simulink model "TST_CoPT_TrqDesCoord"  (R2016b)
settings: Solver=FixedStepDiscrete  StartTime=0.0  StopTime=simTime  FixedStep=sampleTime  RelTol=1e-3
values from neighbouring files (symbols this model uses):
  testCase = 1    [initTST_CoPT_TrqDesCoord_001.m]    (also in initTST_CoPT_TrqDesCoord_002.m = 2; initTST_CoPT_TrqDesCoord_003.m = 3)
libraries: simulink x16, UnitTest_Lib x12
settings Model: Creator=zhengjinyan  LastModifiedBy=zhengjinyan
settings DebuggingCC: SignalRangeChecking=error

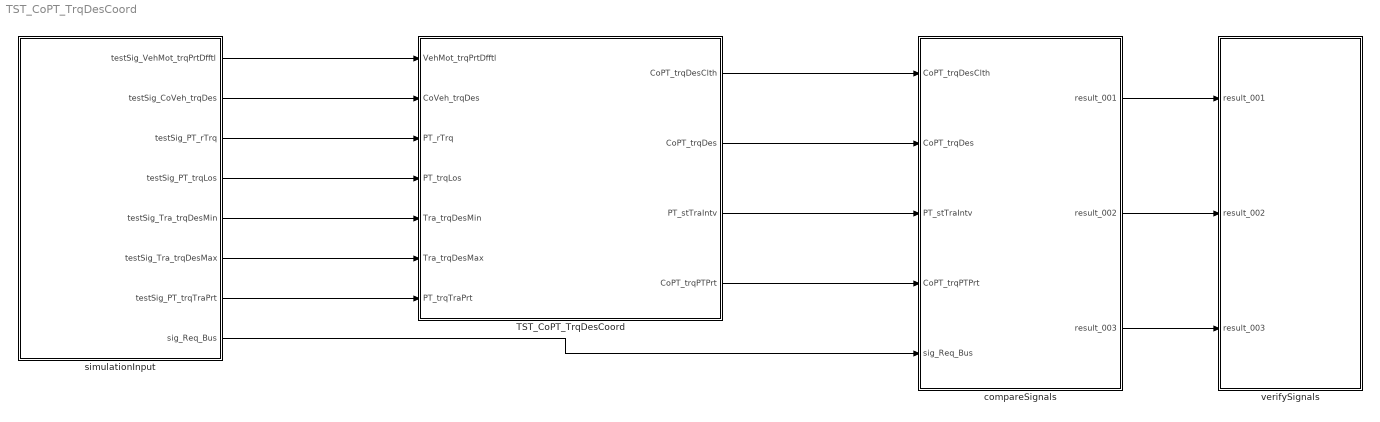
== system TST_CoPT_TrqDesCoord ==
  TST_CoPT_TrqDesCoord : Subsystem
  compareSignals : Subsystem
  simulationInput : Subsystem
  verifySignals : Subsystem
  wires:
  simulationInput/1(testSig_VehMot_trqPrtDfftl) -> TST_CoPT_TrqDesCoord/1(VehMot_trqPrtDfftl)
  simulationInput/2(testSig_CoVeh_trqDes) -> TST_CoPT_TrqDesCoord/2(CoVeh_trqDes)
  simulationInput/3(testSig_PT_rTrq) -> TST_CoPT_TrqDesCoord/3(PT_rTrq)
  simulationInput/4(testSig_PT_trqLos) -> TST_CoPT_TrqDesCoord/4(PT_trqLos)
  simulationInput/5(testSig_Tra_trqDesMin) -> TST_CoPT_TrqDesCoord/5(Tra_trqDesMin)
  simulationInput/6(testSig_Tra_trqDesMax) -> TST_CoPT_TrqDesCoord/6(Tra_trqDesMax)
  simulationInput/7(testSig_PT_trqTraPrt) -> TST_CoPT_TrqDesCoord/7(PT_trqTraPrt)
  TST_CoPT_TrqDesCoord/1(CoPT_trqDesClth) -> compareSignals/1(CoPT_trqDesClth)
  TST_CoPT_TrqDesCoord/2(CoPT_trqDes) -> compareSignals/2(CoPT_trqDes)
  TST_CoPT_TrqDesCoord/3(PT_stTraIntv) -> compareSignals/3(PT_stTraIntv)
  TST_CoPT_TrqDesCoord/4(CoPT_trqPTPrt) -> compareSignals/4(CoPT_trqPTPrt)
  simulationInput/8(sig_Req_Bus) -> compareSignals/5(sig_Req_Bus)
  compareSignals/1(result_001) -> verifySignals/1(result_001)
  compareSignals/2(result_002) -> verifySignals/2(result_002)
  compareSignals/3(result_003) -> verifySignals/3(result_003)

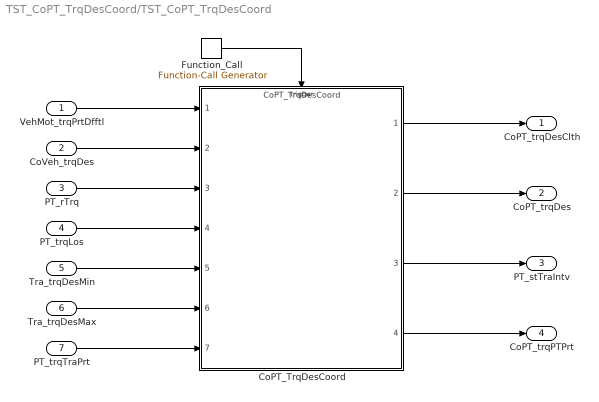
== system TST_CoPT_TrqDesCoord/TST_CoPT_TrqDesCoord ==
  VehMot_trqPrtDfftl : Inport
  CoVeh_trqDes : Inport  Port=2
  PT_rTrq : Inport  Port=3
  PT_trqLos : Inport  Port=4
  Tra_trqDesMin : Inport  Port=5
  Tra_trqDesMax : Inport  Port=6
  PT_trqTraPrt : Inport  Port=7
  CoPT_TrqDesCoord : ModelReference  ModelNameDialog=CoPT_TrqDesCoord  SimulationMode=Normal  ModelReferenceVersion=1.6  TriggerPortName=function  TriggerPortTriggerType=function-call  TriggerPortStatesWhenEnabling=held
  Function_Call : simulink/Ports & Subsystems/Function-Call Generator  sample_time=sampleTime  numberOfIterations=1
  CoPT_trqDesClth : Outport
  CoPT_trqDes : Outport  Port=2
  PT_stTraIntv : Outport  Port=3
  CoPT_trqPTPrt : Outport  Port=4
  wires:
  Function_Call/1 -> CoPT_TrqDesCoord/Trigger
  VehMot_trqPrtDfftl/1 -> CoPT_TrqDesCoord/1
  CoVeh_trqDes/1 -> CoPT_TrqDesCoord/2
  PT_rTrq/1 -> CoPT_TrqDesCoord/3
  PT_trqLos/1 -> CoPT_TrqDesCoord/4
  Tra_trqDesMin/1 -> CoPT_TrqDesCoord/5
  Tra_trqDesMax/1 -> CoPT_TrqDesCoord/6
  PT_trqTraPrt/1 -> CoPT_TrqDesCoord/7
  CoPT_TrqDesCoord/1 -> CoPT_trqDesClth/1
  CoPT_TrqDesCoord/2 -> CoPT_trqDes/1
  CoPT_TrqDesCoord/3 -> PT_stTraIntv/1
  CoPT_TrqDesCoord/4 -> CoPT_trqPTPrt/1

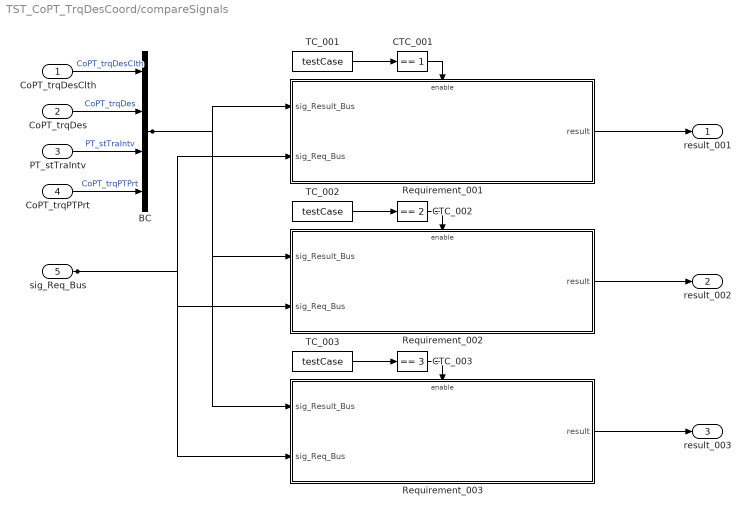
== system TST_CoPT_TrqDesCoord/compareSignals ==
  CoPT_trqDesClth : Inport
  CoPT_trqDes : Inport  Port=2
  PT_stTraIntv : Inport  Port=3
  CoPT_trqPTPrt : Inport  Port=4
  sig_Req_Bus : Inport  Port=5
  BC : BusCreator  Inputs=4
  CTC_001 : simulink/Logic and Bit Operations/Compare To Constant  relop===  const=1  OutDataTypeStr=boolean
  CTC_002 : simulink/Logic and Bit Operations/Compare To Constant  relop===  const=2  OutDataTypeStr=boolean
  CTC_003 : simulink/Logic and Bit Operations/Compare To Constant  relop===  const=3  OutDataTypeStr=boolean
  Requirement_001 : Subsystem
  Requirement_002 : Subsystem
  Requirement_003 : Subsystem
  TC_001 : Constant  Value=testCase
  TC_002 : Constant  Value=testCase
  TC_003 : Constant  Value=testCase
  result_001 : Outport
  result_002 : Outport  Port=2
  result_003 : Outport  Port=3
  wires:
  CoPT_trqDesClth/1 -> BC/1  "CoPT_trqDesClth"
  CoPT_trqDes/1 -> BC/2  "CoPT_trqDes"
  PT_stTraIntv/1 -> BC/3  "PT_stTraIntv"
  CoPT_trqPTPrt/1 -> BC/4  "CoPT_trqPTPrt"
  TC_001/1 -> CTC_001/1
  CTC_001/1 -> Requirement_001/Enable
  sig_Req_Bus/1 -> Requirement_001/2(sig_Req_Bus), Requirement_002/2(sig_Req_Bus), Requirement_003/2(sig_Req_Bus)
  BC/1 -> Requirement_001/1(sig_Result_Bus), Requirement_002/1(sig_Result_Bus), Requirement_003/1(sig_Result_Bus)
  Requirement_001/1(result) -> result_001/1
  TC_002/1 -> CTC_002/1
  CTC_002/1 -> Requirement_002/Enable
  Requirement_002/1(result) -> result_002/1
  TC_003/1 -> CTC_003/1
  CTC_003/1 -> Requirement_003/Enable
  Requirement_003/1(result) -> result_003/1

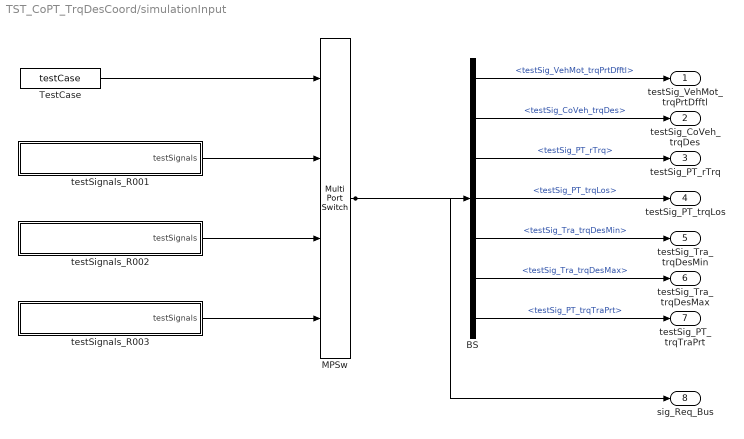
== system TST_CoPT_TrqDesCoord/simulationInput ==
  BS : BusSelector  OutputSignals=testSig_VehMot_trqPrtDfftl,testSig_CoVeh_trqDes,testSig_PT_rTrq,testSig_PT_trqLos,testSig_Tra_trqDesMin,testSig_Tra_trqDesMax,testSig_PT_trqTraPrt
  MPSw : MultiPortSwitch  SaturateOnIntegerOverflow=on  InputSameDT=on
  TestCase : Constant  Value=testCase
  testSignals_R001 : Subsystem
  testSignals_R002 : Subsystem
  testSignals_R003 : Subsystem
  testSig_VehMot_trqPrtDfftl : Outport
  testSig_CoVeh_trqDes : Outport  Port=2
  testSig_PT_rTrq : Outport  Port=3
  testSig_PT_trqLos : Outport  Port=4
  testSig_Tra_trqDesMin : Outport  Port=5
  testSig_Tra_trqDesMax : Outport  Port=6
  testSig_PT_trqTraPrt : Outport  Port=7
  sig_Req_Bus : Outport  Port=8
  wires:
  BS/1 -> testSig_VehMot_trqPrtDfftl/1  "<testSig_VehMot_trqPrtDfftl>"
  BS/2 -> testSig_CoVeh_trqDes/1  "<testSig_CoVeh_trqDes>"
  BS/3 -> testSig_PT_rTrq/1  "<testSig_PT_rTrq>"
  BS/4 -> testSig_PT_trqLos/1  "<testSig_PT_trqLos>"
  BS/5 -> testSig_Tra_trqDesMin/1  "<testSig_Tra_trqDesMin>"
  BS/6 -> testSig_Tra_trqDesMax/1  "<testSig_Tra_trqDesMax>"
  BS/7 -> testSig_PT_trqTraPrt/1  "<testSig_PT_trqTraPrt>"
  MPSw/1 -> BS/1, sig_Req_Bus/1
  TestCase/1 -> MPSw/1
  testSignals_R001/1(testSignals) -> MPSw/2
  testSignals_R002/1(testSignals) -> MPSw/3
  testSignals_R003/1(testSignals) -> MPSw/4

== system TST_CoPT_TrqDesCoord/verifySignals ==
  result_001 : Inport
  result_002 : Inport  Port=2
  result_003 : Inport  Port=3
  Assertion_001 : Assertion  Enabled=off
  Assertion_002 : Assertion  Enabled=off
  Assertion_003 : Assertion  Enabled=off
  wires:
  result_001/1 -> Assertion_001/1
  result_002/1 -> Assertion_002/1
  result_003/1 -> Assertion_003/1

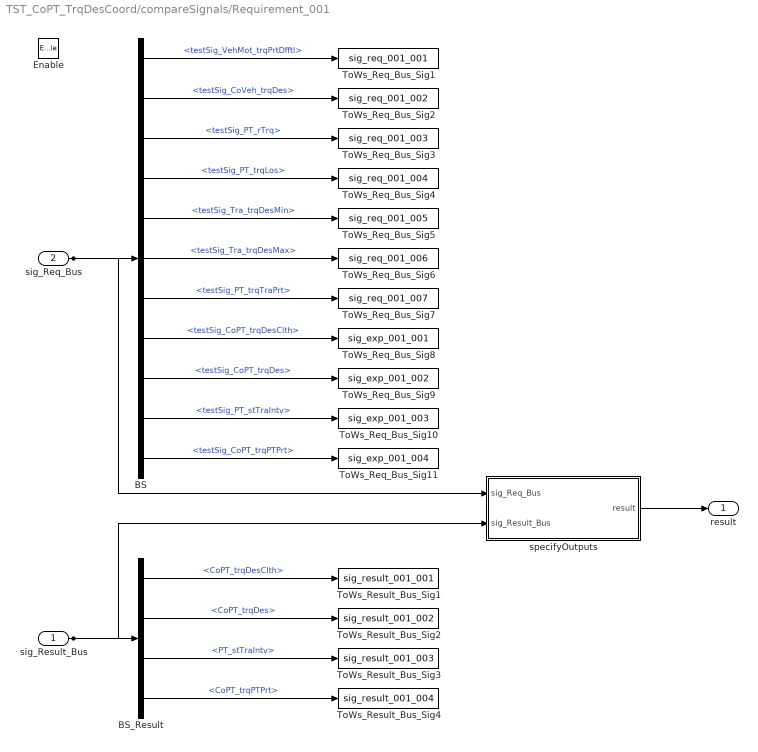
== system TST_CoPT_TrqDesCoord/compareSignals/Requirement_001 ==
  sig_Result_Bus : Inport
  sig_Req_Bus : Inport  Port=2
  Enable : EnablePort
  BS : BusSelector  OutputSignals=testSig_VehMot_trqPrtDfftl,testSig_CoVeh_trqDes,testSig_PT_rTrq,testSig_PT_trqLos,testSig_Tra_trqDesMin,testSig_Tra_trqDesMax,testSig_PT_trqTraPrt,testSig_CoPT_trqDesClth,testSig_CoPT_trqDes,testSig_PT_stTraIntv,testSig_CoPT_trqPTPrt
  BS_Result : BusSelector  OutputSignals=CoPT_trqDesClth,CoPT_trqDes,PT_stTraIntv,CoPT_trqPTPrt
  ToWs_Req_Bus_Sig1 : ToWorkspace  VariableName=sig_req_001_001  SaveFormat=Structure With Time
  ToWs_Req_Bus_Sig10 : ToWorkspace  VariableName=sig_exp_001_003  SaveFormat=Structure With Time
  ToWs_Req_Bus_Sig11 : ToWorkspace  VariableName=sig_exp_001_004  SaveFormat=Structure With Time
  ToWs_Req_Bus_Sig2 : ToWorkspace  VariableName=sig_req_001_002  SaveFormat=Structure With Time
  ToWs_Req_Bus_Sig3 : ToWorkspace  VariableName=sig_req_001_003  SaveFormat=Structure With Time
  ToWs_Req_Bus_Sig4 : ToWorkspace  VariableName=sig_req_001_004  SaveFormat=Structure With Time
  ToWs_Req_Bus_Sig5 : ToWorkspace  VariableName=sig_req_001_005  SaveFormat=Structure With Time
  ToWs_Req_Bus_Sig6 : ToWorkspace  VariableName=sig_req_001_006  SaveFormat=Structure With Time
  ToWs_Req_Bus_Sig7 : ToWorkspace  VariableName=sig_req_001_007  SaveFormat=Structure With Time
  ToWs_Req_Bus_Sig8 : ToWorkspace  VariableName=sig_exp_001_001  SaveFormat=Structure With Time
  ToWs_Req_Bus_Sig9 : ToWorkspace  VariableName=sig_exp_001_002  SaveFormat=Structure With Time
  ToWs_Result_Bus_Sig1 : ToWorkspace  VariableName=sig_result_001_001  SaveFormat=Structure With Time
  ToWs_Result_Bus_Sig2 : ToWorkspace  VariableName=sig_result_001_002  SaveFormat=Structure With Time
  ToWs_Result_Bus_Sig3 : ToWorkspace  VariableName=sig_result_001_003  SaveFormat=Structure With Time
  ToWs_Result_Bus_Sig4 : ToWorkspace  VariableName=sig_result_001_004  SaveFormat=Structure With Time
  specifyOutputs : Subsystem
  result : Outport
  wires:
  sig_Req_Bus/1 -> BS/1, specifyOutputs/1(sig_Req_Bus)
  BS/1 -> ToWs_Req_Bus_Sig1/1  "<testSig_VehMot_trqPrtDfftl>"
  BS/2 -> ToWs_Req_Bus_Sig2/1  "<testSig_CoVeh_trqDes>"
  BS/3 -> ToWs_Req_Bus_Sig3/1  "<testSig_PT_rTrq>"
  BS/4 -> ToWs_Req_Bus_Sig4/1  "<testSig_PT_trqLos>"
  BS/5 -> ToWs_Req_Bus_Sig5/1  "<testSig_Tra_trqDesMin>"
  BS/6 -> ToWs_Req_Bus_Sig6/1  "<testSig_Tra_trqDesMax>"
  BS/7 -> ToWs_Req_Bus_Sig7/1  "<testSig_PT_trqTraPrt>"
  BS/8 -> ToWs_Req_Bus_Sig8/1  "<testSig_CoPT_trqDesClth>"
  BS/9 -> ToWs_Req_Bus_Sig9/1  "<testSig_CoPT_trqDes>"
  BS/10 -> ToWs_Req_Bus_Sig10/1  "<testSig_PT_stTraIntv>"
  BS/11 -> ToWs_Req_Bus_Sig11/1  "<testSig_CoPT_trqPTPrt>"
  sig_Result_Bus/1 -> BS_Result/1, specifyOutputs/2(sig_Result_Bus)
  BS_Result/1 -> ToWs_Result_Bus_Sig1/1  "<CoPT_trqDesClth>"
  BS_Result/2 -> ToWs_Result_Bus_Sig2/1  "<CoPT_trqDes>"
  BS_Result/3 -> ToWs_Result_Bus_Sig3/1  "<PT_stTraIntv>"
  BS_Result/4 -> ToWs_Result_Bus_Sig4/1  "<CoPT_trqPTPrt>"
  specifyOutputs/1(result) -> result/1

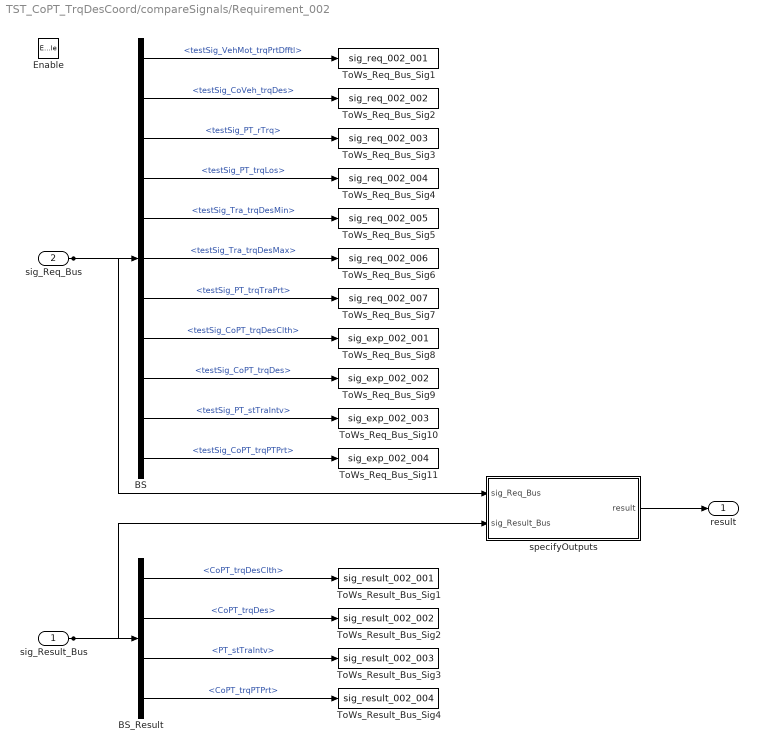
== system TST_CoPT_TrqDesCoord/compareSignals/Requirement_002 ==
  sig_Result_Bus : Inport
  sig_Req_Bus : Inport  Port=2
  Enable : EnablePort
  BS : BusSelector  OutputSignals=testSig_VehMot_trqPrtDfftl,testSig_CoVeh_trqDes,testSig_PT_rTrq,testSig_PT_trqLos,testSig_Tra_trqDesMin,testSig_Tra_trqDesMax,testSig_PT_trqTraPrt,testSig_CoPT_trqDesClth,testSig_CoPT_trqDes,testSig_PT_stTraIntv,testSig_CoPT_trqPTPrt
  BS_Result : BusSelector  OutputSignals=CoPT_trqDesClth,CoPT_trqDes,PT_stTraIntv,CoPT_trqPTPrt
  ToWs_Req_Bus_Sig1 : ToWorkspace  VariableName=sig_req_002_001  SaveFormat=Structure With Time
  ToWs_Req_Bus_Sig10 : ToWorkspace  VariableName=sig_exp_002_003  SaveFormat=Structure With Time
  ToWs_Req_Bus_Sig11 : ToWorkspace  VariableName=sig_exp_002_004  SaveFormat=Structure With Time
  ToWs_Req_Bus_Sig2 : ToWorkspace  VariableName=sig_req_002_002  SaveFormat=Structure With Time
  ToWs_Req_Bus_Sig3 : ToWorkspace  VariableName=sig_req_002_003  SaveFormat=Structure With Time
  ToWs_Req_Bus_Sig4 : ToWorkspace  VariableName=sig_req_002_004  SaveFormat=Structure With Time
  ToWs_Req_Bus_Sig5 : ToWorkspace  VariableName=sig_req_002_005  SaveFormat=Structure With Time
  ToWs_Req_Bus_Sig6 : ToWorkspace  VariableName=sig_req_002_006  SaveFormat=Structure With Time
  ToWs_Req_Bus_Sig7 : ToWorkspace  VariableName=sig_req_002_007  SaveFormat=Structure With Time
  ToWs_Req_Bus_Sig8 : ToWorkspace  VariableName=sig_exp_002_001  SaveFormat=Structure With Time
  ToWs_Req_Bus_Sig9 : ToWorkspace  VariableName=sig_exp_002_002  SaveFormat=Structure With Time
  ToWs_Result_Bus_Sig1 : ToWorkspace  VariableName=sig_result_002_001  SaveFormat=Structure With Time
  ToWs_Result_Bus_Sig2 : ToWorkspace  VariableName=sig_result_002_002  SaveFormat=Structure With Time
  ToWs_Result_Bus_Sig3 : ToWorkspace  VariableName=sig_result_002_003  SaveFormat=Structure With Time
  ToWs_Result_Bus_Sig4 : ToWorkspace  VariableName=sig_result_002_004  SaveFormat=Structure With Time
  specifyOutputs : Subsystem
  result : Outport
  wires:
  sig_Req_Bus/1 -> BS/1, specifyOutputs/1(sig_Req_Bus)
  BS/1 -> ToWs_Req_Bus_Sig1/1  "<testSig_VehMot_trqPrtDfftl>"
  BS/2 -> ToWs_Req_Bus_Sig2/1  "<testSig_CoVeh_trqDes>"
  BS/3 -> ToWs_Req_Bus_Sig3/1  "<testSig_PT_rTrq>"
  BS/4 -> ToWs_Req_Bus_Sig4/1  "<testSig_PT_trqLos>"
  BS/5 -> ToWs_Req_Bus_Sig5/1  "<testSig_Tra_trqDesMin>"
  BS/6 -> ToWs_Req_Bus_Sig6/1  "<testSig_Tra_trqDesMax>"
  BS/7 -> ToWs_Req_Bus_Sig7/1  "<testSig_PT_trqTraPrt>"
  BS/8 -> ToWs_Req_Bus_Sig8/1  "<testSig_CoPT_trqDesClth>"
  BS/9 -> ToWs_Req_Bus_Sig9/1  "<testSig_CoPT_trqDes>"
  BS/10 -> ToWs_Req_Bus_Sig10/1  "<testSig_PT_stTraIntv>"
  BS/11 -> ToWs_Req_Bus_Sig11/1  "<testSig_CoPT_trqPTPrt>"
  sig_Result_Bus/1 -> BS_Result/1, specifyOutputs/2(sig_Result_Bus)
  BS_Result/1 -> ToWs_Result_Bus_Sig1/1  "<CoPT_trqDesClth>"
  BS_Result/2 -> ToWs_Result_Bus_Sig2/1  "<CoPT_trqDes>"
  BS_Result/3 -> ToWs_Result_Bus_Sig3/1  "<PT_stTraIntv>"
  BS_Result/4 -> ToWs_Result_Bus_Sig4/1  "<CoPT_trqPTPrt>"
  specifyOutputs/1(result) -> result/1

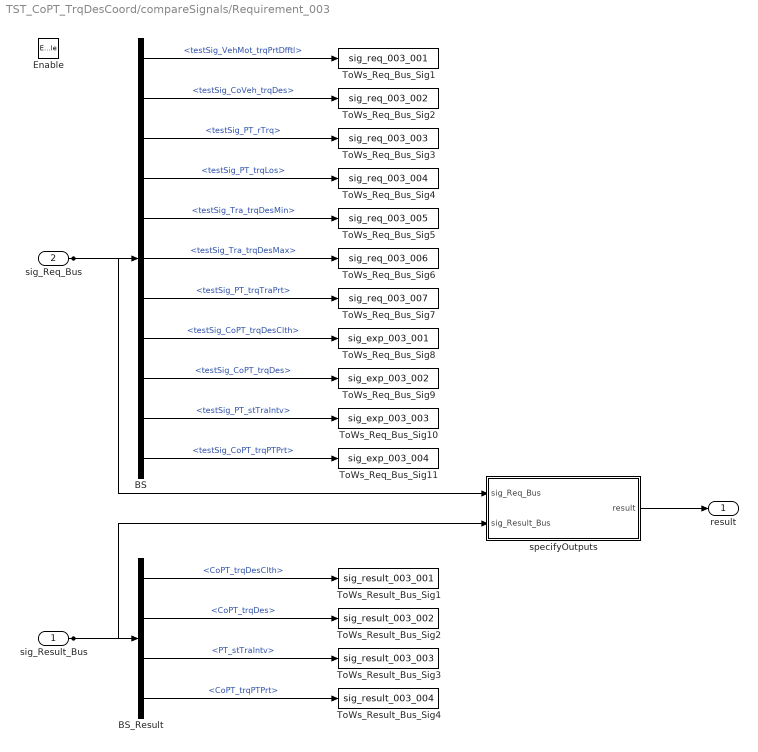
== system TST_CoPT_TrqDesCoord/compareSignals/Requirement_003 ==
  sig_Result_Bus : Inport
  sig_Req_Bus : Inport  Port=2
  Enable : EnablePort
  BS : BusSelector  OutputSignals=testSig_VehMot_trqPrtDfftl,testSig_CoVeh_trqDes,testSig_PT_rTrq,testSig_PT_trqLos,testSig_Tra_trqDesMin,testSig_Tra_trqDesMax,testSig_PT_trqTraPrt,testSig_CoPT_trqDesClth,testSig_CoPT_trqDes,testSig_PT_stTraIntv,testSig_CoPT_trqPTPrt
  BS_Result : BusSelector  OutputSignals=CoPT_trqDesClth,CoPT_trqDes,PT_stTraIntv,CoPT_trqPTPrt
  ToWs_Req_Bus_Sig1 : ToWorkspace  VariableName=sig_req_003_001  SaveFormat=Structure With Time
  ToWs_Req_Bus_Sig10 : ToWorkspace  VariableName=sig_exp_003_003  SaveFormat=Structure With Time
  ToWs_Req_Bus_Sig11 : ToWorkspace  VariableName=sig_exp_003_004  SaveFormat=Structure With Time
  ToWs_Req_Bus_Sig2 : ToWorkspace  VariableName=sig_req_003_002  SaveFormat=Structure With Time
  ToWs_Req_Bus_Sig3 : ToWorkspace  VariableName=sig_req_003_003  SaveFormat=Structure With Time
  ToWs_Req_Bus_Sig4 : ToWorkspace  VariableName=sig_req_003_004  SaveFormat=Structure With Time
  ToWs_Req_Bus_Sig5 : ToWorkspace  VariableName=sig_req_003_005  SaveFormat=Structure With Time
  ToWs_Req_Bus_Sig6 : ToWorkspace  VariableName=sig_req_003_006  SaveFormat=Structure With Time
  ToWs_Req_Bus_Sig7 : ToWorkspace  VariableName=sig_req_003_007  SaveFormat=Structure With Time
  ToWs_Req_Bus_Sig8 : ToWorkspace  VariableName=sig_exp_003_001  SaveFormat=Structure With Time
  ToWs_Req_Bus_Sig9 : ToWorkspace  VariableName=sig_exp_003_002  SaveFormat=Structure With Time
  ToWs_Result_Bus_Sig1 : ToWorkspace  VariableName=sig_result_003_001  SaveFormat=Structure With Time
  ToWs_Result_Bus_Sig2 : ToWorkspace  VariableName=sig_result_003_002  SaveFormat=Structure With Time
  ToWs_Result_Bus_Sig3 : ToWorkspace  VariableName=sig_result_003_003  SaveFormat=Structure With Time
  ToWs_Result_Bus_Sig4 : ToWorkspace  VariableName=sig_result_003_004  SaveFormat=Structure With Time
  specifyOutputs : Subsystem
  result : Outport
  wires:
  sig_Req_Bus/1 -> BS/1, specifyOutputs/1(sig_Req_Bus)
  BS/1 -> ToWs_Req_Bus_Sig1/1  "<testSig_VehMot_trqPrtDfftl>"
  BS/2 -> ToWs_Req_Bus_Sig2/1  "<testSig_CoVeh_trqDes>"
  BS/3 -> ToWs_Req_Bus_Sig3/1  "<testSig_PT_rTrq>"
  BS/4 -> ToWs_Req_Bus_Sig4/1  "<testSig_PT_trqLos>"
  BS/5 -> ToWs_Req_Bus_Sig5/1  "<testSig_Tra_trqDesMin>"
  BS/6 -> ToWs_Req_Bus_Sig6/1  "<testSig_Tra_trqDesMax>"
  BS/7 -> ToWs_Req_Bus_Sig7/1  "<testSig_PT_trqTraPrt>"
  BS/8 -> ToWs_Req_Bus_Sig8/1  "<testSig_CoPT_trqDesClth>"
  BS/9 -> ToWs_Req_Bus_Sig9/1  "<testSig_CoPT_trqDes>"
  BS/10 -> ToWs_Req_Bus_Sig10/1  "<testSig_PT_stTraIntv>"
  BS/11 -> ToWs_Req_Bus_Sig11/1  "<testSig_CoPT_trqPTPrt>"
  sig_Result_Bus/1 -> BS_Result/1, specifyOutputs/2(sig_Result_Bus)
  BS_Result/1 -> ToWs_Result_Bus_Sig1/1  "<CoPT_trqDesClth>"
  BS_Result/2 -> ToWs_Result_Bus_Sig2/1  "<CoPT_trqDes>"
  BS_Result/3 -> ToWs_Result_Bus_Sig3/1  "<PT_stTraIntv>"
  BS_Result/4 -> ToWs_Result_Bus_Sig4/1  "<CoPT_trqPTPrt>"
  specifyOutputs/1(result) -> result/1

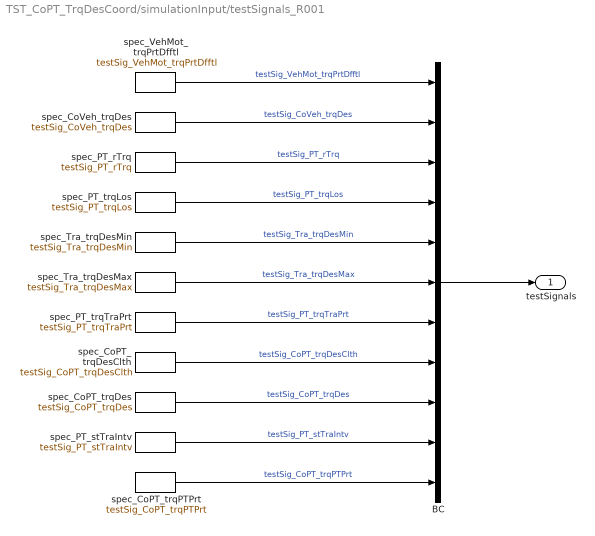
== system TST_CoPT_TrqDesCoord/simulationInput/testSignals_R001 ==
  BC : BusCreator  Inputs=11
  spec_CoPT_trqDes : FromWorkspace  VariableName=testSig_CoPT_trqDes  Interpolate=off  OutputAfterFinalValue=Holding final value
  spec_CoPT_trqDesClth : FromWorkspace  VariableName=testSig_CoPT_trqDesClth  Interpolate=off  OutputAfterFinalValue=Holding final value
  spec_CoPT_trqPTPrt : FromWorkspace  VariableName=testSig_CoPT_trqPTPrt  Interpolate=off  OutputAfterFinalValue=Holding final value
  spec_CoVeh_trqDes : FromWorkspace  VariableName=testSig_CoVeh_trqDes  Interpolate=off  OutputAfterFinalValue=Holding final value
  spec_PT_rTrq : FromWorkspace  VariableName=testSig_PT_rTrq  Interpolate=off  OutputAfterFinalValue=Holding final value
  spec_PT_stTraIntv : FromWorkspace  VariableName=testSig_PT_stTraIntv  Interpolate=off  OutputAfterFinalValue=Holding final value
  spec_PT_trqLos : FromWorkspace  VariableName=testSig_PT_trqLos  Interpolate=off  OutputAfterFinalValue=Holding final value
  spec_PT_trqTraPrt : FromWorkspace  VariableName=testSig_PT_trqTraPrt  Interpolate=off  OutputAfterFinalValue=Holding final value
  spec_Tra_trqDesMax : FromWorkspace  VariableName=testSig_Tra_trqDesMax  Interpolate=off  OutputAfterFinalValue=Holding final value
  spec_Tra_trqDesMin : FromWorkspace  VariableName=testSig_Tra_trqDesMin  Interpolate=off  OutputAfterFinalValue=Holding final value
  spec_VehMot_trqPrtDfftl : FromWorkspace  VariableName=testSig_VehMot_trqPrtDfftl  Interpolate=off  OutputAfterFinalValue=Holding final value
  testSignals : Outport
  wires:
  BC/1 -> testSignals/1
  spec_VehMot_trqPrtDfftl/1 -> BC/1  "testSig_VehMot_trqPrtDfftl"
  spec_CoVeh_trqDes/1 -> BC/2  "testSig_CoVeh_trqDes"
  spec_PT_rTrq/1 -> BC/3  "testSig_PT_rTrq"
  spec_PT_trqLos/1 -> BC/4  "testSig_PT_trqLos"
  spec_Tra_trqDesMin/1 -> BC/5  "testSig_Tra_trqDesMin"
  spec_Tra_trqDesMax/1 -> BC/6  "testSig_Tra_trqDesMax"
  spec_PT_trqTraPrt/1 -> BC/7  "testSig_PT_trqTraPrt"
  spec_CoPT_trqDesClth/1 -> BC/8  "testSig_CoPT_trqDesClth"
  spec_CoPT_trqDes/1 -> BC/9  "testSig_CoPT_trqDes"
  spec_PT_stTraIntv/1 -> BC/10  "testSig_PT_stTraIntv"
  spec_CoPT_trqPTPrt/1 -> BC/11  "testSig_CoPT_trqPTPrt"

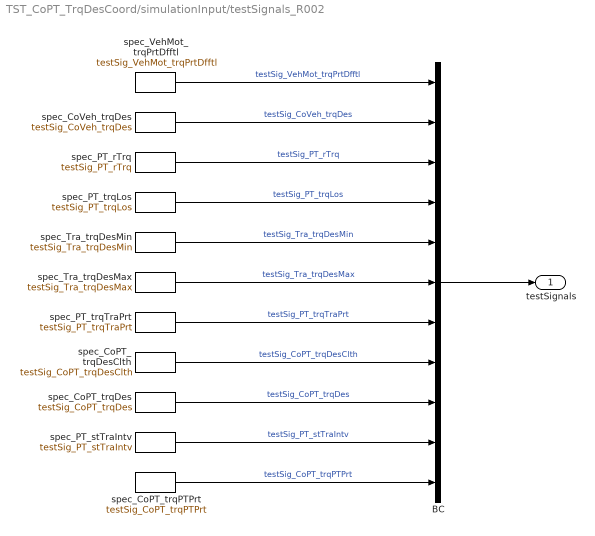
== system TST_CoPT_TrqDesCoord/simulationInput/testSignals_R002 ==
  BC : BusCreator  Inputs=11
  spec_CoPT_trqDes : FromWorkspace  VariableName=testSig_CoPT_trqDes  Interpolate=off  OutputAfterFinalValue=Holding final value
  spec_CoPT_trqDesClth : FromWorkspace  VariableName=testSig_CoPT_trqDesClth  Interpolate=off  OutputAfterFinalValue=Holding final value
  spec_CoPT_trqPTPrt : FromWorkspace  VariableName=testSig_CoPT_trqPTPrt  Interpolate=off  OutputAfterFinalValue=Holding final value
  spec_CoVeh_trqDes : FromWorkspace  VariableName=testSig_CoVeh_trqDes  Interpolate=off  OutputAfterFinalValue=Holding final value
  spec_PT_rTrq : FromWorkspace  VariableName=testSig_PT_rTrq  Interpolate=off  OutputAfterFinalValue=Holding final value
  spec_PT_stTraIntv : FromWorkspace  VariableName=testSig_PT_stTraIntv  Interpolate=off  OutputAfterFinalValue=Holding final value
  spec_PT_trqLos : FromWorkspace  VariableName=testSig_PT_trqLos  Interpolate=off  OutputAfterFinalValue=Holding final value
  spec_PT_trqTraPrt : FromWorkspace  VariableName=testSig_PT_trqTraPrt  Interpolate=off  OutputAfterFinalValue=Holding final value
  spec_Tra_trqDesMax : FromWorkspace  VariableName=testSig_Tra_trqDesMax  Interpolate=off  OutputAfterFinalValue=Holding final value
  spec_Tra_trqDesMin : FromWorkspace  VariableName=testSig_Tra_trqDesMin  Interpolate=off  OutputAfterFinalValue=Holding final value
  spec_VehMot_trqPrtDfftl : FromWorkspace  VariableName=testSig_VehMot_trqPrtDfftl  Interpolate=off  OutputAfterFinalValue=Holding final value
  testSignals : Outport
  wires:
  BC/1 -> testSignals/1
  spec_VehMot_trqPrtDfftl/1 -> BC/1  "testSig_VehMot_trqPrtDfftl"
  spec_CoVeh_trqDes/1 -> BC/2  "testSig_CoVeh_trqDes"
  spec_PT_rTrq/1 -> BC/3  "testSig_PT_rTrq"
  spec_PT_trqLos/1 -> BC/4  "testSig_PT_trqLos"
  spec_Tra_trqDesMin/1 -> BC/5  "testSig_Tra_trqDesMin"
  spec_Tra_trqDesMax/1 -> BC/6  "testSig_Tra_trqDesMax"
  spec_PT_trqTraPrt/1 -> BC/7  "testSig_PT_trqTraPrt"
  spec_CoPT_trqDesClth/1 -> BC/8  "testSig_CoPT_trqDesClth"
  spec_CoPT_trqDes/1 -> BC/9  "testSig_CoPT_trqDes"
  spec_PT_stTraIntv/1 -> BC/10  "testSig_PT_stTraIntv"
  spec_CoPT_trqPTPrt/1 -> BC/11  "testSig_CoPT_trqPTPrt"

== system TST_CoPT_TrqDesCoord/simulationInput/testSignals_R003 ==
  BC : BusCreator  Inputs=11
  spec_CoPT_trqDes : FromWorkspace  VariableName=testSig_CoPT_trqDes  Interpolate=off  OutputAfterFinalValue=Holding final value
  spec_CoPT_trqDesClth : FromWorkspace  VariableName=testSig_CoPT_trqDesClth  Interpolate=off  OutputAfterFinalValue=Holding final value
  spec_CoPT_trqPTPrt : FromWorkspace  VariableName=testSig_CoPT_trqPTPrt  Interpolate=off  OutputAfterFinalValue=Holding final value
  spec_CoVeh_trqDes : FromWorkspace  VariableName=testSig_CoVeh_trqDes  Interpolate=off  OutputAfterFinalValue=Holding final value
  spec_PT_rTrq : FromWorkspace  VariableName=testSig_PT_rTrq  Interpolate=off  OutputAfterFinalValue=Holding final value
  spec_PT_stTraIntv : FromWorkspace  VariableName=testSig_PT_stTraIntv  Interpolate=off  OutputAfterFinalValue=Holding final value
  spec_PT_trqLos : FromWorkspace  VariableName=testSig_PT_trqLos  Interpolate=off  OutputAfterFinalValue=Holding final value
  spec_PT_trqTraPrt : FromWorkspace  VariableName=testSig_PT_trqTraPrt  Interpolate=off  OutputAfterFinalValue=Holding final value
  spec_Tra_trqDesMax : FromWorkspace  VariableName=testSig_Tra_trqDesMax  Interpolate=off  OutputAfterFinalValue=Holding final value
  spec_Tra_trqDesMin : FromWorkspace  VariableName=testSig_Tra_trqDesMin  Interpolate=off  OutputAfterFinalValue=Holding final value
  spec_VehMot_trqPrtDfftl : FromWorkspace  VariableName=testSig_VehMot_trqPrtDfftl  Interpolate=off  OutputAfterFinalValue=Holding final value
  testSignals : Outport
  wires:
  BC/1 -> testSignals/1
  spec_VehMot_trqPrtDfftl/1 -> BC/1  "testSig_VehMot_trqPrtDfftl"
  spec_CoVeh_trqDes/1 -> BC/2  "testSig_CoVeh_trqDes"
  spec_PT_rTrq/1 -> BC/3  "testSig_PT_rTrq"
  spec_PT_trqLos/1 -> BC/4  "testSig_PT_trqLos"
  spec_Tra_trqDesMin/1 -> BC/5  "testSig_Tra_trqDesMin"
  spec_Tra_trqDesMax/1 -> BC/6  "testSig_Tra_trqDesMax"
  spec_PT_trqTraPrt/1 -> BC/7  "testSig_PT_trqTraPrt"
  spec_CoPT_trqDesClth/1 -> BC/8  "testSig_CoPT_trqDesClth"
  spec_CoPT_trqDes/1 -> BC/9  "testSig_CoPT_trqDes"
  spec_PT_stTraIntv/1 -> BC/10  "testSig_PT_stTraIntv"
  spec_CoPT_trqPTPrt/1 -> BC/11  "testSig_CoPT_trqPTPrt"

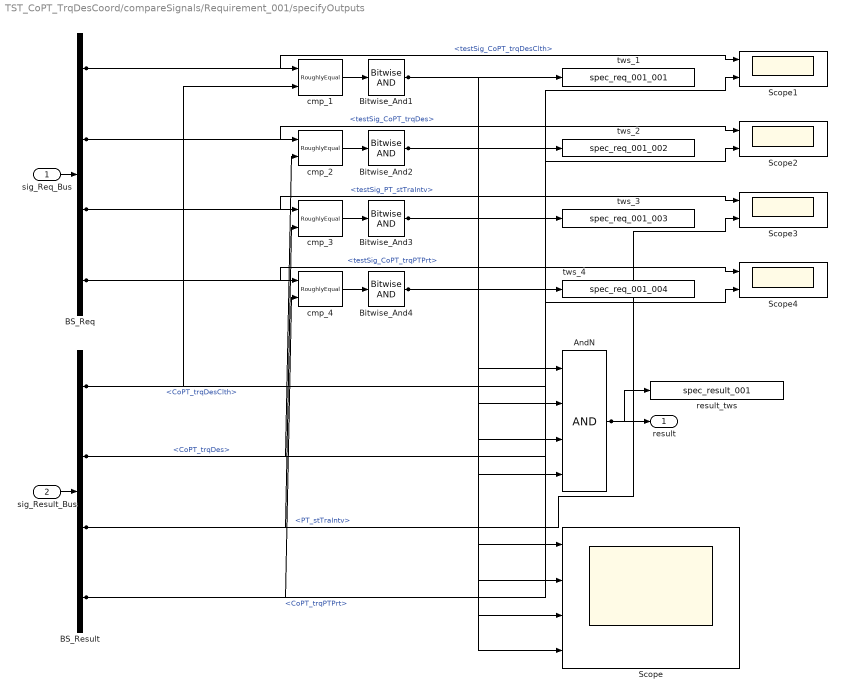
== system TST_CoPT_TrqDesCoord/compareSignals/Requirement_001/specifyOutputs ==
  sig_Req_Bus : Inport
  sig_Result_Bus : Inport  Port=2
  AndN : Logic  Inputs=4
  BS_Req : BusSelector  OutputSignals=testSig_CoPT_trqDesClth,testSig_CoPT_trqDes,testSig_PT_stTraIntv,testSig_CoPT_trqPTPrt
  BS_Result : BusSelector  OutputSignals=CoPT_trqDesClth,CoPT_trqDes,PT_stTraIntv,CoPT_trqPTPrt
  Bitwise_And{1..4} (4 alike) : simulink/Logic and Bit Operations/Bitwise Operator  logicop=AND  UseBitMask=off  BitMask=bin2dec('11011001')  BitMaskRealWorld=Stored Integer
  Scope : Scope  NumInputPorts=4
  Scope{1..4} (4 alike) : Scope  NumInputPorts=2
  cmp_{1..4} (4 alike) : UnitTest_Lib/RoughlyEqual  slope=0.1
  result_tws : ToWorkspace  VariableName=spec_result_001
  tws_1 : ToWorkspace  VariableName=spec_req_001_001
  tws_2 : ToWorkspace  VariableName=spec_req_001_002
  tws_3 : ToWorkspace  VariableName=spec_req_001_003
  tws_4 : ToWorkspace  VariableName=spec_req_001_004
  result : Outport
  wires:
  sig_Req_Bus/1 -> BS_Req/1
  sig_Result_Bus/1 -> BS_Result/1
  AndN/1 -> result/1, result_tws/1
  BS_Req/1 -> cmp_1/1, Scope1/1  "<testSig_CoPT_trqDesClth>"
  BS_Result/1 -> cmp_1/2, Scope1/2  "<CoPT_trqDesClth>"
  cmp_1/1 -> Bitwise_And1/1
  Bitwise_And1/1 -> tws_1/1, AndN/1, Scope/1
  BS_Req/2 -> cmp_2/1, Scope2/1  "<testSig_CoPT_trqDes>"
  BS_Result/2 -> cmp_2/2, Scope2/2  "<CoPT_trqDes>"
  cmp_2/1 -> Bitwise_And2/1
  Bitwise_And2/1 -> tws_2/1, AndN/2, Scope/2
  BS_Req/3 -> cmp_3/1, Scope3/1  "<testSig_PT_stTraIntv>"
  BS_Result/3 -> cmp_3/2, Scope3/2  "<PT_stTraIntv>"
  cmp_3/1 -> Bitwise_And3/1
  Bitwise_And3/1 -> tws_3/1, AndN/3, Scope/3
  BS_Req/4 -> cmp_4/1, Scope4/1  "<testSig_CoPT_trqPTPrt>"
  BS_Result/4 -> cmp_4/2, Scope4/2  "<CoPT_trqPTPrt>"
  cmp_4/1 -> Bitwise_And4/1
  Bitwise_And4/1 -> tws_4/1, AndN/4, Scope/4

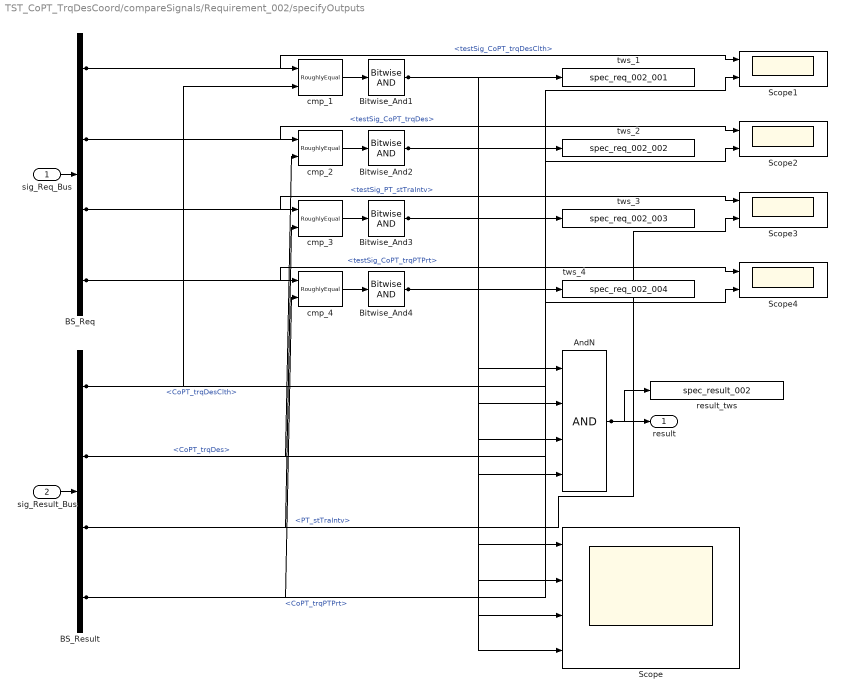
== system TST_CoPT_TrqDesCoord/compareSignals/Requirement_002/specifyOutputs ==
  sig_Req_Bus : Inport
  sig_Result_Bus : Inport  Port=2
  AndN : Logic  Inputs=4
  BS_Req : BusSelector  OutputSignals=testSig_CoPT_trqDesClth,testSig_CoPT_trqDes,testSig_PT_stTraIntv,testSig_CoPT_trqPTPrt
  BS_Result : BusSelector  OutputSignals=CoPT_trqDesClth,CoPT_trqDes,PT_stTraIntv,CoPT_trqPTPrt
  Bitwise_And{1..4} (4 alike) : simulink/Logic and Bit Operations/Bitwise Operator  logicop=AND  UseBitMask=off  BitMask=bin2dec('11011001')  BitMaskRealWorld=Stored Integer
  Scope : Scope  NumInputPorts=4
  Scope{1..4} (4 alike) : Scope  NumInputPorts=2
  cmp_{1..4} (4 alike) : UnitTest_Lib/RoughlyEqual  slope=0.1
  result_tws : ToWorkspace  VariableName=spec_result_002
  tws_1 : ToWorkspace  VariableName=spec_req_002_001
  tws_2 : ToWorkspace  VariableName=spec_req_002_002
  tws_3 : ToWorkspace  VariableName=spec_req_002_003
  tws_4 : ToWorkspace  VariableName=spec_req_002_004
  result : Outport
  wires:
  sig_Req_Bus/1 -> BS_Req/1
  sig_Result_Bus/1 -> BS_Result/1
  AndN/1 -> result/1, result_tws/1
  BS_Req/1 -> cmp_1/1, Scope1/1  "<testSig_CoPT_trqDesClth>"
  BS_Result/1 -> cmp_1/2, Scope1/2  "<CoPT_trqDesClth>"
  cmp_1/1 -> Bitwise_And1/1
  Bitwise_And1/1 -> tws_1/1, AndN/1, Scope/1
  BS_Req/2 -> cmp_2/1, Scope2/1  "<testSig_CoPT_trqDes>"
  BS_Result/2 -> cmp_2/2, Scope2/2  "<CoPT_trqDes>"
  cmp_2/1 -> Bitwise_And2/1
  Bitwise_And2/1 -> tws_2/1, AndN/2, Scope/2
  BS_Req/3 -> cmp_3/1, Scope3/1  "<testSig_PT_stTraIntv>"
  BS_Result/3 -> cmp_3/2, Scope3/2  "<PT_stTraIntv>"
  cmp_3/1 -> Bitwise_And3/1
  Bitwise_And3/1 -> tws_3/1, AndN/3, Scope/3
  BS_Req/4 -> cmp_4/1, Scope4/1  "<testSig_CoPT_trqPTPrt>"
  BS_Result/4 -> cmp_4/2, Scope4/2  "<CoPT_trqPTPrt>"
  cmp_4/1 -> Bitwise_And4/1
  Bitwise_And4/1 -> tws_4/1, AndN/4, Scope/4

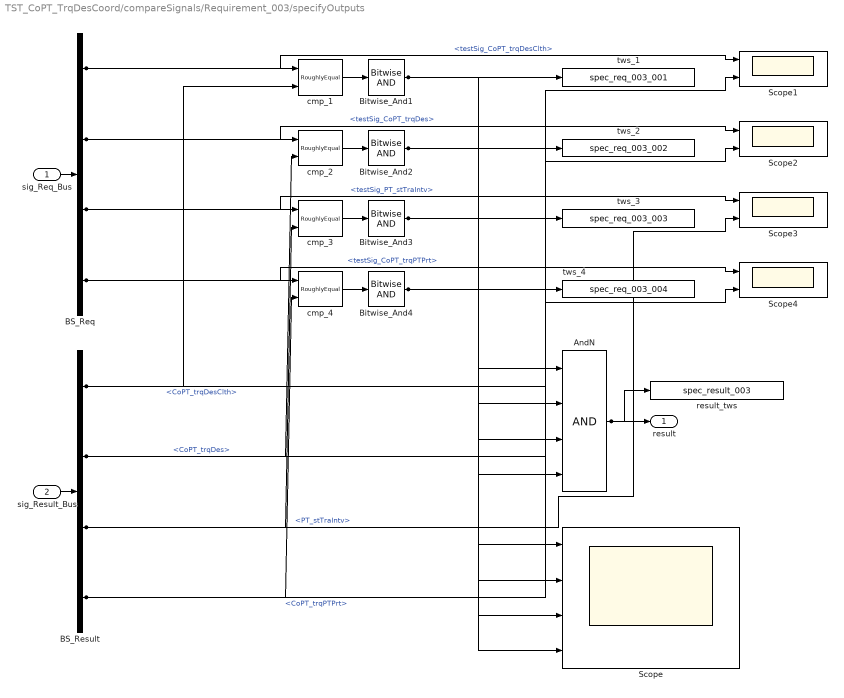
== system TST_CoPT_TrqDesCoord/compareSignals/Requirement_003/specifyOutputs ==
  sig_Req_Bus : Inport
  sig_Result_Bus : Inport  Port=2
  AndN : Logic  Inputs=4
  BS_Req : BusSelector  OutputSignals=testSig_CoPT_trqDesClth,testSig_CoPT_trqDes,testSig_PT_stTraIntv,testSig_CoPT_trqPTPrt
  BS_Result : BusSelector  OutputSignals=CoPT_trqDesClth,CoPT_trqDes,PT_stTraIntv,CoPT_trqPTPrt
  Bitwise_And{1..4} (4 alike) : simulink/Logic and Bit Operations/Bitwise Operator  logicop=AND  UseBitMask=off  BitMask=bin2dec('11011001')  BitMaskRealWorld=Stored Integer
  Scope : Scope  NumInputPorts=4
  Scope{1..4} (4 alike) : Scope  NumInputPorts=2
  cmp_{1..4} (4 alike) : UnitTest_Lib/RoughlyEqual  slope=0.1
  result_tws : ToWorkspace  VariableName=spec_result_003
  tws_1 : ToWorkspace  VariableName=spec_req_003_001
  tws_2 : ToWorkspace  VariableName=spec_req_003_002
  tws_3 : ToWorkspace  VariableName=spec_req_003_003
  tws_4 : ToWorkspace  VariableName=spec_req_003_004
  result : Outport
  wires:
  sig_Req_Bus/1 -> BS_Req/1
  sig_Result_Bus/1 -> BS_Result/1
  AndN/1 -> result/1, result_tws/1
  BS_Req/1 -> cmp_1/1, Scope1/1  "<testSig_CoPT_trqDesClth>"
  BS_Result/1 -> cmp_1/2, Scope1/2  "<CoPT_trqDesClth>"
  cmp_1/1 -> Bitwise_And1/1
  Bitwise_And1/1 -> tws_1/1, AndN/1, Scope/1
  BS_Req/2 -> cmp_2/1, Scope2/1  "<testSig_CoPT_trqDes>"
  BS_Result/2 -> cmp_2/2, Scope2/2  "<CoPT_trqDes>"
  cmp_2/1 -> Bitwise_And2/1
  Bitwise_And2/1 -> tws_2/1, AndN/2, Scope/2
  BS_Req/3 -> cmp_3/1, Scope3/1  "<testSig_PT_stTraIntv>"
  BS_Result/3 -> cmp_3/2, Scope3/2  "<PT_stTraIntv>"
  cmp_3/1 -> Bitwise_And3/1
  Bitwise_And3/1 -> tws_3/1, AndN/3, Scope/3
  BS_Req/4 -> cmp_4/1, Scope4/1  "<testSig_CoPT_trqPTPrt>"
  BS_Result/4 -> cmp_4/2, Scope4/2  "<CoPT_trqPTPrt>"
  cmp_4/1 -> Bitwise_And4/1
  Bitwise_And4/1 -> tws_4/1, AndN/4, Scope/4
